simulink model "Ch2CSTROpenLoop_Sys"  (R2014b)
settings: Solver=ode45  StartTime=0.0  StopTime=10.0  RelTol=1e-5
values from neighbouring files (symbols this model uses):
  C_Afeed = 10    [Ch2CSTRClosedLoop.m]    (also in Ch2CSTRClosedLoopRobustness.m; Ch2CSTROpenLoop.m)
  C_Afeed_Change = -5    [Ch2CSTRClosedLoop.m]    (also in Ch2CSTRClosedLoopRobustness.m = 10; Ch2CSTROpenLoop.m = -10)
  C_Afeed_instant = 10    [Ch2CSTRClosedLoop.m]    (also in Ch2CSTRClosedLoopRobustness.m = 2; Ch2CSTROpenLoop.m)
  Fr_Change = -10    [Ch2CSTRClosedLoop.m]    (also in Ch2CSTRClosedLoopRobustness.m = 0; Ch2CSTROpenLoop.m = 20)
  Fr_in = 60    [Ch2CSTRClosedLoop.m]    (also in Ch2CSTRClosedLoopRobustness.m; Ch2CSTROpenLoop.m)
  Fr_instant = 20    [Ch2CSTRClosedLoop.m]    (also in Ch2CSTRClosedLoopRobustness.m = 2; Ch2CSTROpenLoop.m = 2)
settings Model: Creator=rvilanova  LastModifiedBy=rvilanova
settings DebuggingCC: SolverPrmCheckMsg=none

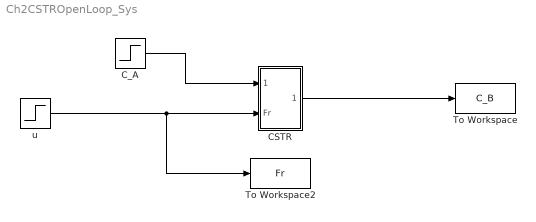
== system Ch2CSTROpenLoop_Sys ==
  "CSTR " : Subsystem
  C_A : Step  Time=C_Afeed_instant  Before=C_Afeed  After=C_Afeed*(1+C_Afeed_Change/100)  SampleTime=0
  To Workspace : ToWorkspace  VariableName=C_B  SaveFormat=Timeseries  SampleTime=-1
  To Workspace2 : ToWorkspace  VariableName=Fr  SaveFormat=Timeseries  SampleTime=-1
  u : Step  Time=Fr_instant  Before=Fr_in  After=Fr_in*(1+Fr_Change/100)  SampleTime=0
  wires:
  u/1 -> To Workspace2/1, "CSTR "/2(Fr)
  "CSTR "/1(C_B) -> To Workspace/1
  C_A/1 -> "CSTR "/1(C_A)

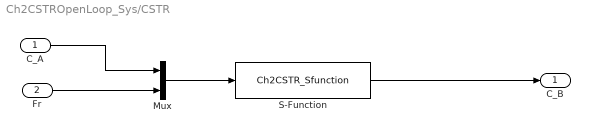
== system Ch2CSTROpenLoop_Sys/CSTR  ==
  C_A : Inport
  Fr : Inport  Port=2
  Mux : Mux  Inputs=2
  S-Function : S-Function  FunctionName=Ch2CSTR_Sfunction  Parameters=C_Ao, C_Bo  EnableBusSupport=off
  C_B : Outport
  wires:
  S-Function/1 -> C_B/1
  Mux/1 -> S-Function/1
  Fr/1 -> Mux/2
  C_A/1 -> Mux/1
